simulink model "uni_bi_polar_SPWM"  (R2023a)
settings: Solver=VariableStepDiscrete  StartTime=0.0  StopTime=.1  RelTol=1e-3
libraries: spsMosfetLib x8, simulink x3, spsDCVoltageSourceLib x2, spsSeriesRLCBranchLib x2, spsVoltageMeasurementLib x2, spspowerguiLib x1
settings Model: Creator=Blu-Ray  LastModifiedBy=Blu-Ray
settings DebuggingCC: UnconnectedInputMsg=warning  UnconnectedOutputMsg=warning  UnconnectedLineMsg=warning
settings ModelReferenceCC: EnableRefExpFcnMdlSchedulingChecks=on
settings RTWCC: DLArmComputeVersion=19.05

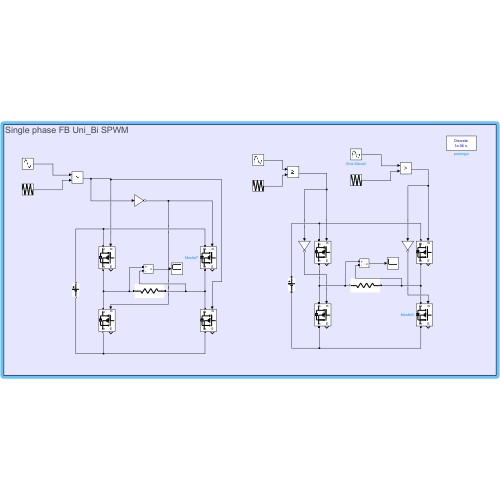
[thumbnail: Simulink's stored preview of the top-level diagram]
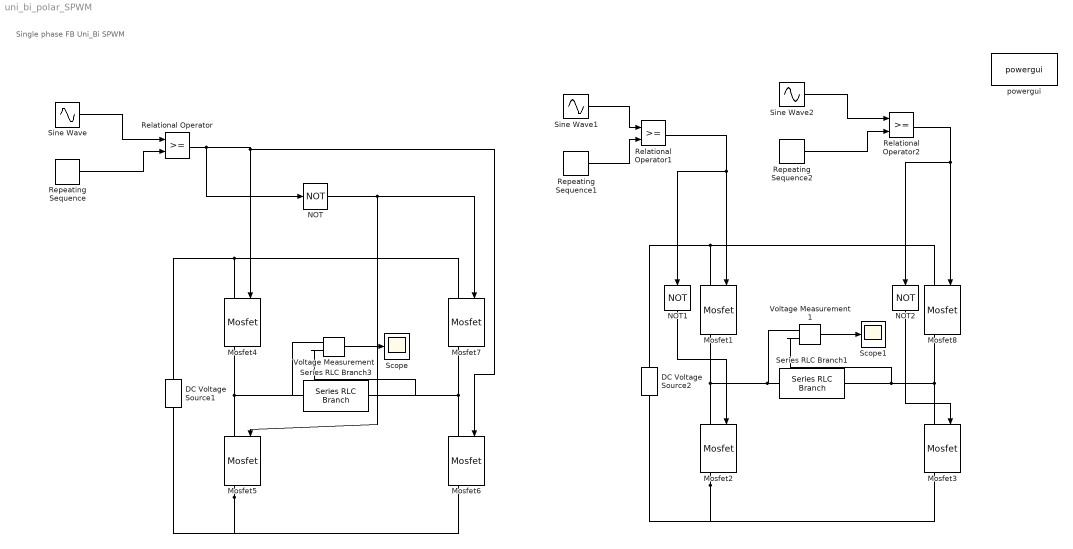
== system uni_bi_polar_SPWM ==
  note: Single phase FB Uni_Bi SPWM
  DC Voltage Source1 : spsDCVoltageSourceLib/DC Voltage Source  Amplitude=100  Measurements=None
  DC Voltage Source2 : spsDCVoltageSourceLib/DC Voltage Source  Amplitude=100  Measurements=None
  Mosfet{1..8} (8 alike) : spsMosfetLib/Mosfet  Ron=0.1  Lon=0  Rd=0.01  Vfd=0  IC=0  Rs=1e5  Cs=inf  Measurements=on
  NOT : Logic  Operator=NOT  IconShape=distinctive  AllPortsSameDT=off  OutDataTypeStr=boolean
  NOT1 : Logic  Operator=NOT  IconShape=distinctive  AllPortsSameDT=off  OutDataTypeStr=boolean
  NOT2 : Logic  Operator=NOT  IconShape=distinctive  AllPortsSameDT=off  OutDataTypeStr=boolean
  Relational Operator : RelationalOperator  OutDataTypeStr=boolean  RndMeth=Simplest  InputSameDT=off
  Relational Operator1 : RelationalOperator  OutDataTypeStr=boolean  RndMeth=Simplest  InputSameDT=off
  Relational Operator2 : RelationalOperator  OutDataTypeStr=boolean  RndMeth=Simplest  InputSameDT=off
  Repeating Sequence : simulink/Sources/Repeating Sequence  rep_seq_t=[0 (1/5050)/4 (1/5050)/2 (3/5050)/4 (1/5050)]  rep_seq_y=[0 1 0 -1 0 ]
  Repeating Sequence1 : simulink/Sources/Repeating Sequence  rep_seq_t=[0 (1/5050)/4 (1/5050)/2 (3/5050)/4 (1/5050)]  rep_seq_y=[0 1 0 -1 0 ]
  Repeating Sequence2 : simulink/Sources/Repeating Sequence  rep_seq_t=[0 (1/5050)/4 (1/5050)/2 (3/5050)/4 (1/5050)]  rep_seq_y=[0 1 0 -1 0 ]
  Scope : Scope
  Scope1 : Scope
  Series RLC Branch1 : spsSeriesRLCBranchLib/Series RLC Branch  LConnTagsString=__new0  RConnTagsString=__new0  BranchType=R  Resistance=10  Inductance=1e-3  SetiL0=off  InitialCurrent=0  Capacitance=1e-6  Setx0=off  InitialVoltage=0  Measurements=None
  Series RLC Branch3 : spsSeriesRLCBranchLib/Series RLC Branch  LConnTagsString=__new0  RConnTagsString=__new0  BranchType=R  Resistance=10  Inductance=1e-3  SetiL0=off  InitialCurrent=0  Capacitance=1e-6  Setx0=off  InitialVoltage=0  Measurements=None
  Sine Wave : Sin  Amplitude=.95  Frequency=2*50*pi  SampleTime=0
  Sine Wave1 : Sin  Amplitude=.95  Frequency=2*50*pi  SampleTime=0
  Sine Wave2 : Sin  Amplitude=.95  Frequency=2*50*pi  Phase=pi  SampleTime=0
  Voltage Measurement : spsVoltageMeasurementLib/Voltage Measurement  PhasorSimulation=off  OutputType=Complex  PSBequivalent=0
  Voltage Measurement1 : spsVoltageMeasurementLib/Voltage Measurement  PhasorSimulation=off  OutputType=Complex  PSBequivalent=0
  powergui : spspowerguiLib/powergui  Priority=1  SimulationMode=Discrete  SampleTime=1e-6  frequency=60  Iterations=50  frequencyindice=0  Pbase=100e6  ErrMax=1e-4  UnitsV=kV  UnitsW=MW  buscounter=0  FunctionMessages=off  echomessages=off  EnableUseOfTLC=off  CurrentSourceSwitches=off  DisableSnubberDevices=off  DisableRonSwitches=off  DisableVfSwitches=off  DisplayEquations=off  AutomaticDiscreteSolvers=off  SolverType=Tustin/Backward Euler (TBE)  Interpol=off  ExternalGateDelay=off  methode=off  Ts=100  x0status=blocks  SPID=on  SwTol=0  HookPort=off  NonlinearTolerance=1e-4  nMaxIteration=100  ContinueOnMaxIteration=off  RestoreLinks=warning  ResistiveCurrentMeasurement=off  Frange=[0:2:500]  Ylog=off  Xlog=on  ShowGrid=off  save=off  variable=ZData  structure=0  ZoomFFT=off  StartTime=0.0  cycles=1  DisplayStyle=1  fundamental=60  FreqAxis=off  MaxFrequency=1000  frequencyindicesteady=1  RmsSteady=1  display=off
  wires:
  Sine Wave/1 -> Relational Operator/1
  Repeating Sequence/1 -> Relational Operator/2
  Voltage Measurement/1 -> Scope/1
  Relational Operator/1 -> NOT/1, Mosfet6/1, Mosfet4/1
  NOT/1 -> Mosfet5/1, Mosfet7/1
  Relational Operator1/1 -> NOT1/1, Mosfet1/1
  Voltage Measurement1/1 -> Scope1/1
  Repeating Sequence1/1 -> Relational Operator1/2
  Sine Wave1/1 -> Relational Operator1/1
  NOT1/1 -> Mosfet2/1
  NOT2/1 -> Mosfet3/1
  Sine Wave2/1 -> Relational Operator2/1
  Repeating Sequence2/1 -> Relational Operator2/2
  Relational Operator2/1 -> NOT2/1, Mosfet8/1
  connections:
  DC Voltage Source1/RConn1 -- Mosfet4/LConn1 -- Mosfet7/LConn1
  Mosfet7/RConn1 -- Voltage Measurement/LConn2 -- Series RLC Branch3/LConn1 -- Mosfet6/LConn1
  Mosfet5/RConn1 -- DC Voltage Source1/LConn1 -- Mosfet6/RConn1
  Mosfet4/RConn1 -- Voltage Measurement/LConn1 -- Series RLC Branch3/RConn1 -- Mosfet5/LConn1
  DC Voltage Source2/RConn1 -- Mosfet8/LConn1 -- Mosfet1/LConn1
  Voltage Measurement1/LConn2 -- Series RLC Branch1/LConn1 -- Mosfet8/RConn1 -- Mosfet3/LConn1
  Mosfet2/RConn1 -- Mosfet3/RConn1 -- DC Voltage Source2/LConn1
  Voltage Measurement1/LConn1 -- Series RLC Branch1/RConn1 -- Mosfet1/RConn1 -- Mosfet2/LConn1
